simulink model "untitled"  (R2018b)
settings: Solver=ode15s  StartTime=0.0  StopTime=50  MaxStep=0.1  RelTol=1e-3
values from neighbouring files (symbols this model uses):
  F = [         1, 2, 3, 1;         1, 3, 4, 1;         1, 2, 5, 1;         1, 5, 4, 1;         2, 3, 6, 2;         3, 4, 6, 3;         2, 5, 6, 2;         4, 5, 6, 4;         6, 15, 16, 6;         7, 8, 9, 10;         11, 12, 13, 14;         ]    [drawVehicle.m]    (also in draw_runway.m)
  q = uu(11)    [drawVehicle.m]    (also in forceee.m; plotmavstatevariables.m = 180/pi*uu(11); plotresults.m = 180/pi*uu(11))
  r = uu(12)    [drawVehicle.m]    (also in forceee.m; plotmavstatevariables.m = 180/pi*uu(12); plotresults.m = 180/pi*uu(12))
undefined symbols (not defined in the file or in its folder): Light, MIL
libraries: simulink_extras x3, aerolibwind2 x2, sharedtransform x1
settings Model: Creator=xinyizhao  LastModifiedBy=xinyizhao

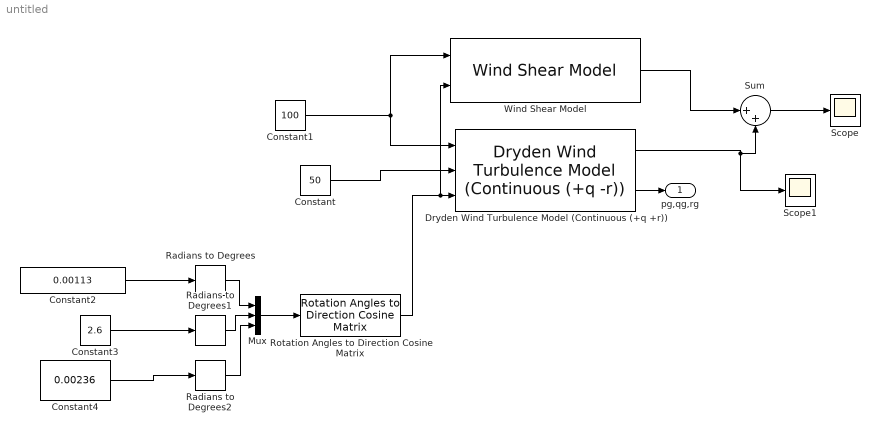
== system untitled ==
  Constant : Constant  Value=50
  Constant1 : Constant  Value=100
  Constant2 : Constant  Value=0.00113
  Constant3 : Constant  Value=2.6
  Constant4 : Constant  Value=0.00236
  Dryden Wind Turbulence Model (Continuous (+q +r)) : aerolibwind2/Dryden Wind Turbulence Model  (Continuous (+q -r))  units=Metric (MKS)  spec=MIL-F-8785C  model=Continuous Dryden (+q +r)  W20=5  Wdeg=0  TurbProb=10^-2 - Light  L_high=533.4  Wingspan=P.b  ts=0.1  Seed=[23341 23342 23343 23344]  T_on=on
      settings: SourceProductName=Aerospace Blockset
  Mux : Mux  Inputs=3
  Radians to Degrees : simulink_extras/Transformations/Radians to Degrees
  Radians to Degrees1 : simulink_extras/Transformations/Radians to Degrees
  Radians to Degrees2 : simulink_extras/Transformations/Radians to Degrees
  Rotation Angles to Direction Cosine Matrix : sharedtransform/Rotation Angles to Direction Cosine Matrix  rotationOrder=ZYX  aMode=aMode
      settings: SourceProductBaseCode=AE
  Scope : Scope
  Scope1 : Scope
  Sum : Sum  Inputs=|++  SaturateOnIntegerOverflow=on  InputSameDT=on  OutDataTypeStr=Inherit: Same as first input
  Wind Shear Model : aerolibwind2/Wind Shear Model  units=Metric (MKS)  phase=Category C - Terminal Flight Phase  W_20=5  Wdeg=0
      settings: SourceProductName=Aerospace Blockset
  pg,qg,rg : Outport  Unit=rad/s
  wires:
  Sum/1 -> Scope/1
  Dryden Wind Turbulence Model (Continuous (+q +r))/2 -> pg,qg,rg/1
  Constant/1 -> Dryden Wind Turbulence Model (Continuous (+q +r))/2
  Constant1/1 -> Dryden Wind Turbulence Model (Continuous (+q +r))/1, Wind Shear Model/1
  Wind Shear Model/1 -> Sum/1
  Radians to Degrees/1 -> Mux/1
  Radians to Degrees1/1 -> Mux/2
  Radians to Degrees2/1 -> Mux/3
  Constant2/1 -> Radians to Degrees/1
  Constant3/1 -> Radians to Degrees1/1
  Constant4/1 -> Radians to Degrees2/1
  Mux/1 -> Rotation Angles to Direction Cosine Matrix/1
  Rotation Angles to Direction Cosine Matrix/1 -> Dryden Wind Turbulence Model (Continuous (+q +r))/3, Wind Shear Model/2
  Dryden Wind Turbulence Model (Continuous (+q +r))/1 -> Sum/2, Scope1/1
